simulink model "ASM_Traffic_V2X_Complete_Model_2"  (R2019a)
settings: Solver=ode1  StartTime=SIM.tstart.v  StopTime=Inf  FixedStep=SIM.StepSize.v  RelTol=1e-3
PostLoadFcn:
  | if any(exist('dsrtsu_mdlpostloadfcn', 'file') ~= 0), dsrtsu_mdlpostloadfcn('Execute', bdroot); end
  | try, asm_mdl_postloadfcn(bdroot, 'UpdateModel', 2200); catch, disp(lasterr); end,
undefined symbols (not defined in the file): _SensorPnts_1, _SensorPnts_13, _SensorPnts_17, _SensorPnts_21, _SensorPnts_25, _SensorPnts_29, _SensorPnts_33, _SensorPnts_37, _SensorPnts_41, _SensorPnts_45, _SensorPnts_49, _SensorPnts_5, _SensorPnts_53, _SensorPnts_57, _SensorPnts_9, _to_, CPT, G5A, ITS, MDL, rad, s_to_rpm, SIM
libraries: simulink x169, ASM_VehicleDynamics_lib x126, ASM_Traffic_lib x83, ASM_Utils_lib x49, mdbs x45, ASM_Environment_lib x17, dspindex x12, dsaV2xLibraryAux x10, dsmpblib x6, dsaV2xAsn1Library x4, dsaV2xLibrary x4, ASM_BrakeHydraulics_lib x4
(part 28 of 36)

== system ASM_Traffic_V2X_Complete_Model_2/MDLUserInterface/MotionDeskInterface/MOTION_DESK_INTERFACE/Traffic_Animation/Fellows_Animation/Fellow_11 ==
  Transform_In : Inport
  Pos_x_Fellows[m] : Inport  Port=2
  Pos_y_Fellows[m] : Inport  Port=3
  Pos_z_Fellows[m] : Inport  Port=4
  Angle_Roll_Fellows[deg] : Inport  Port=5
  Angle_Pitch_Fellows[deg] : Inport  Port=6
  Angle_Yaw_Fellows[deg] : Inport  Port=7
  Flag_FellowUsed : Inport  Port=8
  Constant : Constant  Value=11
  MD_Object : mdbs/MD_Object  strObjId=18  strObjName=Fellow_11  strBlockType=OBJ  bGUIEventOK=0
      settings: SourceProductName=dSPACE MotionDesk Blockset
  Mux : Mux  Inputs=3
  Mux1 : Mux  Inputs=3
  Mux3 : Mux  Inputs=3
  Selector{1..7} (7 alike) : Selector  InputPortWidth=MDL.Traffic.MaxNumFellows.v  IndexOptions=Index vector (port)  Indices=[1 3]  OutputSizes=1
  Terminator : Terminator
  wires:
  Pos_x_Fellows[m]/1 -> Selector1/1
  Pos_y_Fellows[m]/1 -> Selector2/1
  Pos_z_Fellows[m]/1 -> Selector3/1
  Angle_Roll_Fellows[deg]/1 -> Selector4/1
  Angle_Pitch_Fellows[deg]/1 -> Selector5/1
  Angle_Yaw_Fellows[deg]/1 -> Selector7/1
  Selector3/1 -> Mux/3
  Selector2/1 -> Mux/2
  Selector1/1 -> Mux/1
  Constant/1 -> Selector6/2, Selector7/2, Selector5/2, Selector4/2, Selector3/2, Selector2/2, Selector1/2
  Flag_FellowUsed/1 -> Selector6/1
  Mux1/1 -> MD_Object/3
  Mux3/1 -> MD_Object/4
  Transform_In/1 -> MD_Object/1
  Mux/1 -> MD_Object/2
  Selector6/1 -> Mux3/2, Mux3/3, Mux3/1
  MD_Object/1 -> Terminator/1
  Selector5/1 -> Mux1/2
  Selector7/1 -> Mux1/1
  Selector4/1 -> Mux1/3

== system ASM_Traffic_V2X_Complete_Model_2/MDLUserInterface/MotionDeskInterface/MOTION_DESK_INTERFACE/Traffic_Animation/Fellows_Animation/Fellow_12 ==
  Transform_In : Inport
  Pos_x_Fellows[m] : Inport  Port=2
  Pos_y_Fellows[m] : Inport  Port=3
  Pos_z_Fellows[m] : Inport  Port=4
  Angle_Roll_Fellows[deg] : Inport  Port=5
  Angle_Pitch_Fellows[deg] : Inport  Port=6
  Angle_Yaw_Fellows[deg] : Inport  Port=7
  Flag_FellowUsed : Inport  Port=8
  Constant : Constant  Value=12
  MD_Object : mdbs/MD_Object  strObjId=19  strObjName=Fellow_12  strBlockType=OBJ  bGUIEventOK=0
      settings: SourceProductName=dSPACE MotionDesk Blockset
  Mux : Mux  Inputs=3
  Mux1 : Mux  Inputs=3
  Mux3 : Mux  Inputs=3
  Selector{1..7} (7 alike) : Selector  InputPortWidth=MDL.Traffic.MaxNumFellows.v  IndexOptions=Index vector (port)  Indices=[1 3]  OutputSizes=1
  Terminator : Terminator
  wires:
  Pos_x_Fellows[m]/1 -> Selector1/1
  Pos_y_Fellows[m]/1 -> Selector2/1
  Pos_z_Fellows[m]/1 -> Selector3/1
  Angle_Roll_Fellows[deg]/1 -> Selector4/1
  Angle_Pitch_Fellows[deg]/1 -> Selector5/1
  Angle_Yaw_Fellows[deg]/1 -> Selector7/1
  Selector3/1 -> Mux/3
  Selector2/1 -> Mux/2
  Selector1/1 -> Mux/1
  Constant/1 -> Selector7/2, Selector6/2, Selector5/2, Selector4/2, Selector3/2, Selector2/2, Selector1/2
  Flag_FellowUsed/1 -> Selector6/1
  Mux1/1 -> MD_Object/3
  Mux3/1 -> MD_Object/4
  Transform_In/1 -> MD_Object/1
  Mux/1 -> MD_Object/2
  Selector6/1 -> Mux3/2, Mux3/3, Mux3/1
  MD_Object/1 -> Terminator/1
  Selector5/1 -> Mux1/2
  Selector7/1 -> Mux1/1
  Selector4/1 -> Mux1/3

== system ASM_Traffic_V2X_Complete_Model_2/MDLUserInterface/MotionDeskInterface/MOTION_DESK_INTERFACE/Traffic_Animation/Fellows_Animation/Fellow_13 ==
  Transform_In : Inport
  Pos_x_Fellows[m] : Inport  Port=2
  Pos_y_Fellows[m] : Inport  Port=3
  Pos_z_Fellows[m] : Inport  Port=4
  Angle_Roll_Fellows[deg] : Inport  Port=5
  Angle_Pitch_Fellows[deg] : Inport  Port=6
  Angle_Yaw_Fellows[deg] : Inport  Port=7
  Flag_FellowUsed : Inport  Port=8
  Constant : Constant  Value=13
  MD_Object : mdbs/MD_Object  strObjId=20  strObjName=Fellow_13  strBlockType=OBJ  bGUIEventOK=0
      settings: SourceProductName=dSPACE MotionDesk Blockset
  Mux : Mux  Inputs=3
  Mux1 : Mux  Inputs=3
  Mux3 : Mux  Inputs=3
  Selector{1..7} (7 alike) : Selector  InputPortWidth=MDL.Traffic.MaxNumFellows.v  IndexOptions=Index vector (port)  Indices=[1 3]  OutputSizes=1
  Terminator : Terminator
  wires:
  Pos_x_Fellows[m]/1 -> Selector1/1
  Pos_y_Fellows[m]/1 -> Selector2/1
  Pos_z_Fellows[m]/1 -> Selector3/1
  Angle_Roll_Fellows[deg]/1 -> Selector4/1
  Angle_Pitch_Fellows[deg]/1 -> Selector5/1
  Angle_Yaw_Fellows[deg]/1 -> Selector7/1
  Selector3/1 -> Mux/3
  Selector2/1 -> Mux/2
  Selector1/1 -> Mux/1
  Constant/1 -> Selector1/2, Selector6/2, Selector7/2, Selector5/2, Selector4/2, Selector3/2, Selector2/2
  Flag_FellowUsed/1 -> Selector6/1
  Mux1/1 -> MD_Object/3
  Mux3/1 -> MD_Object/4
  Transform_In/1 -> MD_Object/1
  Mux/1 -> MD_Object/2
  Selector6/1 -> Mux3/3, Mux3/2, Mux3/1
  MD_Object/1 -> Terminator/1
  Selector5/1 -> Mux1/2
  Selector7/1 -> Mux1/1
  Selector4/1 -> Mux1/3

== system ASM_Traffic_V2X_Complete_Model_2/MDLUserInterface/MotionDeskInterface/MOTION_DESK_INTERFACE/Traffic_Animation/Fellows_Animation/Fellow_14 ==
  Transform_In : Inport
  Pos_x_Fellows[m] : Inport  Port=2
  Pos_y_Fellows[m] : Inport  Port=3
  Pos_z_Fellows[m] : Inport  Port=4
  Angle_Roll_Fellows[deg] : Inport  Port=5
  Angle_Pitch_Fellows[deg] : Inport  Port=6
  Angle_Yaw_Fellows[deg] : Inport  Port=7
  Flag_FellowUsed : Inport  Port=8
  Constant : Constant  Value=14
  MD_Object : mdbs/MD_Object  strObjId=21  strObjName=Fellow_14  strBlockType=OBJ  bGUIEventOK=0
      settings: SourceProductName=dSPACE MotionDesk Blockset
  Mux : Mux  Inputs=3
  Mux1 : Mux  Inputs=3
  Mux3 : Mux  Inputs=3
  Selector{1..7} (7 alike) : Selector  InputPortWidth=MDL.Traffic.MaxNumFellows.v  IndexOptions=Index vector (port)  Indices=[1 3]  OutputSizes=1
  Terminator : Terminator
  wires:
  Pos_x_Fellows[m]/1 -> Selector1/1
  Pos_y_Fellows[m]/1 -> Selector2/1
  Pos_z_Fellows[m]/1 -> Selector3/1
  Angle_Roll_Fellows[deg]/1 -> Selector4/1
  Angle_Pitch_Fellows[deg]/1 -> Selector5/1
  Angle_Yaw_Fellows[deg]/1 -> Selector7/1
  Selector3/1 -> Mux/3
  Selector2/1 -> Mux/2
  Selector1/1 -> Mux/1
  Constant/1 -> Selector1/2, Selector6/2, Selector7/2, Selector5/2, Selector4/2, Selector3/2, Selector2/2
  Flag_FellowUsed/1 -> Selector6/1
  Mux1/1 -> MD_Object/3
  Mux3/1 -> MD_Object/4
  Transform_In/1 -> MD_Object/1
  Mux/1 -> MD_Object/2
  Selector6/1 -> Mux3/2, Mux3/3, Mux3/1
  MD_Object/1 -> Terminator/1
  Selector5/1 -> Mux1/2
  Selector7/1 -> Mux1/1
  Selector4/1 -> Mux1/3

== system ASM_Traffic_V2X_Complete_Model_2/MDLUserInterface/MotionDeskInterface/MOTION_DESK_INTERFACE/Traffic_Animation/Fellows_Animation/Fellow_15 ==
  Transform_In : Inport
  Pos_x_Fellows[m] : Inport  Port=2
  Pos_y_Fellows[m] : Inport  Port=3
  Pos_z_Fellows[m] : Inport  Port=4
  Angle_Roll_Fellows[deg] : Inport  Port=5
  Angle_Pitch_Fellows[deg] : Inport  Port=6
  Angle_Yaw_Fellows[deg] : Inport  Port=7
  Flag_FellowUsed : Inport  Port=8
  Constant : Constant  Value=15
  MD_Object : mdbs/MD_Object  strObjId=22  strObjName=Fellow_15  strBlockType=OBJ  bGUIEventOK=0
      settings: SourceProductName=dSPACE MotionDesk Blockset
  Mux : Mux  Inputs=3
  Mux1 : Mux  Inputs=3
  Mux3 : Mux  Inputs=3
  Selector{1..7} (7 alike) : Selector  InputPortWidth=MDL.Traffic.MaxNumFellows.v  IndexOptions=Index vector (port)  Indices=[1 3]  OutputSizes=1
  Terminator : Terminator
  wires:
  Pos_x_Fellows[m]/1 -> Selector1/1
  Pos_y_Fellows[m]/1 -> Selector2/1
  Pos_z_Fellows[m]/1 -> Selector3/1
  Angle_Roll_Fellows[deg]/1 -> Selector4/1
  Angle_Pitch_Fellows[deg]/1 -> Selector5/1
  Angle_Yaw_Fellows[deg]/1 -> Selector7/1
  Selector3/1 -> Mux/3
  Selector2/1 -> Mux/2
  Selector1/1 -> Mux/1
  Constant/1 -> Selector7/2, Selector6/2, Selector5/2, Selector4/2, Selector3/2, Selector2/2, Selector1/2
  Flag_FellowUsed/1 -> Selector6/1
  Mux1/1 -> MD_Object/3
  Mux3/1 -> MD_Object/4
  Transform_In/1 -> MD_Object/1
  Mux/1 -> MD_Object/2
  Selector6/1 -> Mux3/2, Mux3/3, Mux3/1
  MD_Object/1 -> Terminator/1
  Selector5/1 -> Mux1/2
  Selector7/1 -> Mux1/1
  Selector4/1 -> Mux1/3

== system ASM_Traffic_V2X_Complete_Model_2/MDLUserInterface/MotionDeskInterface/MOTION_DESK_INTERFACE/Traffic_Animation/Fellows_Animation/Fellow_2 ==
  Transform_In : Inport
  Pos_x_Fellows[m] : Inport  Port=2
  Pos_y_Fellows[m] : Inport  Port=3
  Pos_z_Fellows[m] : Inport  Port=4
  Angle_Roll_Fellows[deg] : Inport  Port=5
  Angle_Pitch_Fellows[deg] : Inport  Port=6
  Angle_Yaw_Fellows[deg] : Inport  Port=7
  Flag_FellowUsed : Inport  Port=8
  Constant : Constant  Value=2
  MD_Object : mdbs/MD_Object  strObjId=9  strObjName=Fellow_02  strBlockType=OBJ  bGUIEventOK=0
      settings: SourceProductName=dSPACE MotionDesk Blockset
  Mux : Mux  Inputs=3
  Mux1 : Mux  Inputs=3
  Mux3 : Mux  Inputs=3
  Selector{1..7} (7 alike) : Selector  InputPortWidth=MDL.Traffic.MaxNumFellows.v  IndexOptions=Index vector (port)  Indices=[1 3]  OutputSizes=1
  Terminator : Terminator
  wires:
  Pos_x_Fellows[m]/1 -> Selector1/1
  Pos_y_Fellows[m]/1 -> Selector2/1
  Pos_z_Fellows[m]/1 -> Selector3/1
  Angle_Roll_Fellows[deg]/1 -> Selector4/1
  Angle_Pitch_Fellows[deg]/1 -> Selector5/1
  Angle_Yaw_Fellows[deg]/1 -> Selector7/1
  Selector3/1 -> Mux/3
  Selector2/1 -> Mux/2
  Selector1/1 -> Mux/1
  Constant/1 -> Selector7/2, Selector6/2, Selector5/2, Selector4/2, Selector3/2, Selector2/2, Selector1/2
  Flag_FellowUsed/1 -> Selector6/1
  Mux3/1 -> MD_Object/4
  Transform_In/1 -> MD_Object/1
  Mux/1 -> MD_Object/2
  Mux1/1 -> MD_Object/3
  Selector6/1 -> Mux3/2, Mux3/3, Mux3/1
  MD_Object/1 -> Terminator/1
  Selector5/1 -> Mux1/2
  Selector7/1 -> Mux1/1
  Selector4/1 -> Mux1/3

== system ASM_Traffic_V2X_Complete_Model_2/MDLUserInterface/MotionDeskInterface/MOTION_DESK_INTERFACE/Traffic_Animation/Fellows_Animation/Fellow_3 ==
  Transform_In : Inport
  Pos_x_Fellows[m] : Inport  Port=2
  Pos_y_Fellows[m] : Inport  Port=3
  Pos_z_Fellows[m] : Inport  Port=4
  Angle_Roll_Fellows[deg] : Inport  Port=5
  Angle_Pitch_Fellows[deg] : Inport  Port=6
  Angle_Yaw_Fellows[deg] : Inport  Port=7
  Flag_FellowUsed : Inport  Port=8
  Constant : Constant  Value=3
  MD_Object : mdbs/MD_Object  strObjId=10  strObjName=Fellow_03  strBlockType=OBJ  bGUIEventOK=0
      settings: SourceProductName=dSPACE MotionDesk Blockset
  Mux : Mux  Inputs=3
  Mux1 : Mux  Inputs=3
  Mux3 : Mux  Inputs=3
  Selector{1..7} (7 alike) : Selector  InputPortWidth=MDL.Traffic.MaxNumFellows.v  IndexOptions=Index vector (port)  Indices=[1 3]  OutputSizes=1
  Terminator : Terminator
  wires:
  Selector4/1 -> Mux1/3
  Selector7/1 -> Mux1/1
  Selector5/1 -> Mux1/2
  MD_Object/1 -> Terminator/1
  Selector6/1 -> Mux3/1, Mux3/3, Mux3/2
  Mux1/1 -> MD_Object/3
  Mux/1 -> MD_Object/2
  Transform_In/1 -> MD_Object/1
  Mux3/1 -> MD_Object/4
  Flag_FellowUsed/1 -> Selector6/1
  Constant/1 -> Selector6/2, Selector7/2, Selector5/2, Selector4/2, Selector3/2, Selector2/2, Selector1/2
  Selector1/1 -> Mux/1
  Selector2/1 -> Mux/2
  Selector3/1 -> Mux/3
  Angle_Yaw_Fellows[deg]/1 -> Selector7/1
  Angle_Pitch_Fellows[deg]/1 -> Selector5/1
  Angle_Roll_Fellows[deg]/1 -> Selector4/1
  Pos_z_Fellows[m]/1 -> Selector3/1
  Pos_y_Fellows[m]/1 -> Selector2/1
  Pos_x_Fellows[m]/1 -> Selector1/1

== system ASM_Traffic_V2X_Complete_Model_2/MDLUserInterface/MotionDeskInterface/MOTION_DESK_INTERFACE/Traffic_Animation/Fellows_Animation/Fellow_4 ==
  Transform_In : Inport
  Pos_x_Fellows[m] : Inport  Port=2
  Pos_y_Fellows[m] : Inport  Port=3
  Pos_z_Fellows[m] : Inport  Port=4
  Angle_Roll_Fellows[deg] : Inport  Port=5
  Angle_Pitch_Fellows[deg] : Inport  Port=6
  Angle_Yaw_Fellows[deg] : Inport  Port=7
  Flag_FellowUsed : Inport  Port=8
  Constant : Constant  Value=4
  MD_Object : mdbs/MD_Object  strObjId=11  strObjName=Fellow_04  strBlockType=OBJ  bGUIEventOK=0
      settings: SourceProductName=dSPACE MotionDesk Blockset
  Mux : Mux  Inputs=3
  Mux1 : Mux  Inputs=3
  Mux3 : Mux  Inputs=3
  Selector{1..7} (7 alike) : Selector  InputPortWidth=MDL.Traffic.MaxNumFellows.v  IndexOptions=Index vector (port)  Indices=[1 3]  OutputSizes=1
  Terminator : Terminator
  wires:
  Pos_x_Fellows[m]/1 -> Selector1/1
  Pos_y_Fellows[m]/1 -> Selector2/1
  Pos_z_Fellows[m]/1 -> Selector3/1
  Angle_Roll_Fellows[deg]/1 -> Selector4/1
  Angle_Pitch_Fellows[deg]/1 -> Selector5/1
  Angle_Yaw_Fellows[deg]/1 -> Selector7/1
  Selector3/1 -> Mux/3
  Selector2/1 -> Mux/2
  Selector1/1 -> Mux/1
  Constant/1 -> Selector7/2, Selector6/2, Selector5/2, Selector4/2, Selector3/2, Selector2/2, Selector1/2
  Flag_FellowUsed/1 -> Selector6/1
  Mux3/1 -> MD_Object/4
  Transform_In/1 -> MD_Object/1
  Mux/1 -> MD_Object/2
  Mux1/1 -> MD_Object/3
  Selector6/1 -> Mux3/2, Mux3/3, Mux3/1
  MD_Object/1 -> Terminator/1
  Selector5/1 -> Mux1/2
  Selector7/1 -> Mux1/1
  Selector4/1 -> Mux1/3

== system ASM_Traffic_V2X_Complete_Model_2/MDLUserInterface/MotionDeskInterface/MOTION_DESK_INTERFACE/Traffic_Animation/Fellows_Animation/Fellow_5 ==
  Transform_In : Inport
  Pos_x_Fellows[m] : Inport  Port=2
  Pos_y_Fellows[m] : Inport  Port=3
  Pos_z_Fellows[m] : Inport  Port=4
  Angle_Roll_Fellows[deg] : Inport  Port=5
  Angle_Pitch_Fellows[deg] : Inport  Port=6
  Angle_Yaw_Fellows[deg] : Inport  Port=7
  Flag_FellowUsed : Inport  Port=8
  Constant : Constant  Value=5
  MD_Object : mdbs/MD_Object  strObjId=12  strObjName=Fellow_05  strBlockType=OBJ  bGUIEventOK=0
      settings: SourceProductName=dSPACE MotionDesk Blockset
  Mux : Mux  Inputs=3
  Mux1 : Mux  Inputs=3
  Mux3 : Mux  Inputs=3
  Selector{1..7} (7 alike) : Selector  InputPortWidth=MDL.Traffic.MaxNumFellows.v  IndexOptions=Index vector (port)  Indices=[1 3]  OutputSizes=1
  Terminator : Terminator
  wires:
  Pos_x_Fellows[m]/1 -> Selector1/1
  Pos_y_Fellows[m]/1 -> Selector2/1
  Pos_z_Fellows[m]/1 -> Selector3/1
  Angle_Roll_Fellows[deg]/1 -> Selector4/1
  Angle_Pitch_Fellows[deg]/1 -> Selector5/1
  Angle_Yaw_Fellows[deg]/1 -> Selector7/1
  Selector3/1 -> Mux/3
  Selector2/1 -> Mux/2
  Selector1/1 -> Mux/1
  Constant/1 -> Selector7/2, Selector6/2, Selector5/2, Selector4/2, Selector3/2, Selector2/2, Selector1/2
  Flag_FellowUsed/1 -> Selector6/1
  Mux1/1 -> MD_Object/3
  Mux3/1 -> MD_Object/4
  Transform_In/1 -> MD_Object/1
  Mux/1 -> MD_Object/2
  Selector6/1 -> Mux3/2, Mux3/3, Mux3/1
  MD_Object/1 -> Terminator/1
  Selector5/1 -> Mux1/2
  Selector7/1 -> Mux1/1
  Selector4/1 -> Mux1/3

== system ASM_Traffic_V2X_Complete_Model_2/MDLUserInterface/MotionDeskInterface/MOTION_DESK_INTERFACE/Traffic_Animation/Fellows_Animation/Fellow_6 ==
  Transform_In : Inport
  Pos_x_Fellows[m] : Inport  Port=2
  Pos_y_Fellows[m] : Inport  Port=3
  Pos_z_Fellows[m] : Inport  Port=4
  Angle_Roll_Fellows[deg] : Inport  Port=5
  Angle_Pitch_Fellows[deg] : Inport  Port=6
  Angle_Yaw_Fellows[deg] : Inport  Port=7
  Flag_FellowUsed : Inport  Port=8
  Constant : Constant  Value=6
  MD_Object : mdbs/MD_Object  strObjId=13  strObjName=Fellow_06  strBlockType=OBJ  bGUIEventOK=0
      settings: SourceProductName=dSPACE MotionDesk Blockset
  Mux : Mux  Inputs=3
  Mux1 : Mux  Inputs=3
  Mux3 : Mux  Inputs=3
  Selector{1..7} (7 alike) : Selector  InputPortWidth=MDL.Traffic.MaxNumFellows.v  IndexOptions=Index vector (port)  Indices=[1 3]  OutputSizes=1
  Terminator : Terminator
  wires:
  Pos_x_Fellows[m]/1 -> Selector1/1
  Pos_y_Fellows[m]/1 -> Selector2/1
  Pos_z_Fellows[m]/1 -> Selector3/1
  Angle_Roll_Fellows[deg]/1 -> Selector4/1
  Angle_Pitch_Fellows[deg]/1 -> Selector5/1
  Angle_Yaw_Fellows[deg]/1 -> Selector7/1
  Selector3/1 -> Mux/3
  Selector2/1 -> Mux/2
  Selector1/1 -> Mux/1
  Constant/1 -> Selector6/2, Selector7/2, Selector5/2, Selector4/2, Selector3/2, Selector2/2, Selector1/2
  Flag_FellowUsed/1 -> Selector6/1
  Mux1/1 -> MD_Object/3
  Mux3/1 -> MD_Object/4
  Transform_In/1 -> MD_Object/1
  Mux/1 -> MD_Object/2
  Selector6/1 -> Mux3/2, Mux3/3, Mux3/1
  MD_Object/1 -> Terminator/1
  Selector5/1 -> Mux1/2
  Selector7/1 -> Mux1/1
  Selector4/1 -> Mux1/3

== system ASM_Traffic_V2X_Complete_Model_2/MDLUserInterface/MotionDeskInterface/MOTION_DESK_INTERFACE/Traffic_Animation/Fellows_Animation/Fellow_7 ==
  Transform_In : Inport
  Pos_x_Fellows[m] : Inport  Port=2
  Pos_y_Fellows[m] : Inport  Port=3
  Pos_z_Fellows[m] : Inport  Port=4
  Angle_Roll_Fellows[deg] : Inport  Port=5
  Angle_Pitch_Fellows[deg] : Inport  Port=6
  Angle_Yaw_Fellows[deg] : Inport  Port=7
  Flag_FellowUsed : Inport  Port=8
  Constant : Constant  Value=7
  MD_Object : mdbs/MD_Object  strObjId=14  strObjName=Fellow_07  strBlockType=OBJ  bGUIEventOK=0
      settings: SourceProductName=dSPACE MotionDesk Blockset
  Mux : Mux  Inputs=3
  Mux1 : Mux  Inputs=3
  Mux3 : Mux  Inputs=3
  Selector{1..7} (7 alike) : Selector  InputPortWidth=MDL.Traffic.MaxNumFellows.v  IndexOptions=Index vector (port)  Indices=[1 3]  OutputSizes=1
  Terminator : Terminator
  wires:
  Pos_x_Fellows[m]/1 -> Selector1/1
  Pos_y_Fellows[m]/1 -> Selector2/1
  Pos_z_Fellows[m]/1 -> Selector3/1
  Angle_Roll_Fellows[deg]/1 -> Selector4/1
  Angle_Pitch_Fellows[deg]/1 -> Selector5/1
  Angle_Yaw_Fellows[deg]/1 -> Selector7/1
  Selector3/1 -> Mux/3
  Selector2/1 -> Mux/2
  Selector1/1 -> Mux/1
  Constant/1 -> Selector1/2, Selector7/2, Selector6/2, Selector5/2, Selector4/2, Selector3/2, Selector2/2
  Flag_FellowUsed/1 -> Selector6/1
  Mux1/1 -> MD_Object/3
  Mux3/1 -> MD_Object/4
  Transform_In/1 -> MD_Object/1
  Mux/1 -> MD_Object/2
  Selector6/1 -> Mux3/2, Mux3/3, Mux3/1
  MD_Object/1 -> Terminator/1
  Selector5/1 -> Mux1/2
  Selector7/1 -> Mux1/1
  Selector4/1 -> Mux1/3

== system ASM_Traffic_V2X_Complete_Model_2/MDLUserInterface/MotionDeskInterface/MOTION_DESK_INTERFACE/Traffic_Animation/Fellows_Animation/Fellow_8 ==
  Transform_In : Inport
  Pos_x_Fellows[m] : Inport  Port=2
  Pos_y_Fellows[m] : Inport  Port=3
  Pos_z_Fellows[m] : Inport  Port=4
  Angle_Roll_Fellows[deg] : Inport  Port=5
  Angle_Pitch_Fellows[deg] : Inport  Port=6
  Angle_Yaw_Fellows[deg] : Inport  Port=7
  Flag_FellowUsed : Inport  Port=8
  Constant : Constant  Value=8
  MD_Object : mdbs/MD_Object  strObjId=15  strObjName=Fellow_08  strBlockType=OBJ  bGUIEventOK=0
      settings: SourceProductName=dSPACE MotionDesk Blockset
  Mux : Mux  Inputs=3
  Mux1 : Mux  Inputs=3
  Mux3 : Mux  Inputs=3
  Selector{1..7} (7 alike) : Selector  InputPortWidth=MDL.Traffic.MaxNumFellows.v  IndexOptions=Index vector (port)  Indices=[1 3]  OutputSizes=1
  Terminator : Terminator
  wires:
  Pos_x_Fellows[m]/1 -> Selector1/1
  Pos_y_Fellows[m]/1 -> Selector2/1
  Pos_z_Fellows[m]/1 -> Selector3/1
  Angle_Roll_Fellows[deg]/1 -> Selector4/1
  Angle_Pitch_Fellows[deg]/1 -> Selector5/1
  Angle_Yaw_Fellows[deg]/1 -> Selector7/1
  Selector3/1 -> Mux/3
  Selector2/1 -> Mux/2
  Selector1/1 -> Mux/1
  Constant/1 -> Selector7/2, Selector6/2, Selector5/2, Selector4/2, Selector3/2, Selector2/2, Selector1/2
  Flag_FellowUsed/1 -> Selector6/1
  Mux1/1 -> MD_Object/3
  Mux3/1 -> MD_Object/4
  Transform_In/1 -> MD_Object/1
  Mux/1 -> MD_Object/2
  Selector6/1 -> Mux3/2, Mux3/3, Mux3/1
  MD_Object/1 -> Terminator/1
  Selector5/1 -> Mux1/2
  Selector7/1 -> Mux1/1
  Selector4/1 -> Mux1/3

== system ASM_Traffic_V2X_Complete_Model_2/MDLUserInterface/MotionDeskInterface/MOTION_DESK_INTERFACE/Traffic_Animation/Fellows_Animation/Fellow_9 ==
  Transform_In : Inport
  Pos_x_Fellows[m] : Inport  Port=2
  Pos_y_Fellows[m] : Inport  Port=3
  Pos_z_Fellows[m] : Inport  Port=4
  Angle_Roll_Fellows[deg] : Inport  Port=5
  Angle_Pitch_Fellows[deg] : Inport  Port=6
  Angle_Yaw_Fellows[deg] : Inport  Port=7
  Flag_FellowUsed : Inport  Port=8
  Constant : Constant  Value=9
  MD_Object : mdbs/MD_Object  strObjId=16  strObjName=Fellow_09  strBlockType=OBJ  bGUIEventOK=0
      settings: SourceProductName=dSPACE MotionDesk Blockset
  Mux : Mux  Inputs=3
  Mux1 : Mux  Inputs=3
  Mux3 : Mux  Inputs=3
  Selector{1..7} (7 alike) : Selector  InputPortWidth=MDL.Traffic.MaxNumFellows.v  IndexOptions=Index vector (port)  Indices=[1 3]  OutputSizes=1
  Terminator : Terminator
  wires:
  Pos_x_Fellows[m]/1 -> Selector1/1
  Pos_y_Fellows[m]/1 -> Selector2/1
  Pos_z_Fellows[m]/1 -> Selector3/1
  Angle_Roll_Fellows[deg]/1 -> Selector4/1
  Angle_Pitch_Fellows[deg]/1 -> Selector5/1
  Angle_Yaw_Fellows[deg]/1 -> Selector7/1
  Selector3/1 -> Mux/3
  Selector2/1 -> Mux/2
  Selector1/1 -> Mux/1
  Constant/1 -> Selector1/2, Selector6/2, Selector7/2, Selector5/2, Selector4/2, Selector3/2, Selector2/2
  Flag_FellowUsed/1 -> Selector6/1
  Mux1/1 -> MD_Object/3
  Mux3/1 -> MD_Object/4
  Transform_In/1 -> MD_Object/1
  Mux/1 -> MD_Object/2
  Selector6/1 -> Mux3/2, Mux3/3, Mux3/1
  MD_Object/1 -> Terminator/1
  Selector5/1 -> Mux1/2
  Selector7/1 -> Mux1/1
  Selector4/1 -> Mux1/3

== system ASM_Traffic_V2X_Complete_Model_2/MDLUserInterface/MotionDeskInterface/MOTION_DESK_INTERFACE/Traffic_Animation/Sensors_Animation/Sensor_Points ==
  Sw_Sensor_Animation[] : Inport
  Transform_In : Inport  Port=2
  Sensors_Signals : Inport  Port=3
  Bus Selector1 : BusSelector  OutputSignals=Object_Sensor_3D,Object_Sensor_2D,TrafficSign_Sensor_Dyn,Line_Sensor.Line_Sensor_1.Pos_Road_Lane_Animation_CoorSys_E,Line_Sensor.Line_Sensor_1.Pos_Road_Shape_Line_Animation_CoorSys_E,Line_Sensor.Line_Sensor_1.Pos_Road_Shape_ContObj_Animation_CoorSys_E,Line_Sensor.Line_Sensor_1.Pos_Junction_Border_Animation_CoorSys_E,Line_Sensor.Line_Sensor_1.Pos_Junction_Shape_Line_Animation_CoorSys_E,Line_Sensor.Line_Sensor_1.Pos_Junction_Shape_ContObj_Animation_CoorSys_E
  Line_Sensor_Junction_Border_Points : Subsystem
  Line_Sensor_Junction_Shape_ContObj_Points : Subsystem
  Line_Sensor_Junction_Shape_Line_Points : Subsystem
  Line_Sensor_Road_Lane_Points : Subsystem
  Line_Sensor_Road_Shape_ContObj_Points : Subsystem
  Line_Sensor_Road_Shape_Line_Points : Subsystem
  Multiport Switch : MultiPortSwitch  Inputs=11
  Object_Sensor_2D_Points : Subsystem
  Object_Sensor_3D_CustomPoints : Subsystem
  Object_Sensor_3D_Points : Subsystem
  Object_Sensor_3D_RadarEffect_Points : Subsystem
  Saturation : Saturate  UpperLimit=11  LowerLimit=1
  Sensor_Points : Subsystem
  Sensor_Selector : Constant
  Traffic_Sign_Sensor_Points : Subsystem
  wires:
  Sensor_Selector/1 -> Object_Sensor_3D_Points/2(Sensor_Selector), Object_Sensor_3D_CustomPoints/2(Sensor_Selector), Object_Sensor_3D_RadarEffect_Points/2(Sensor_Selector)
  Object_Sensor_3D_CustomPoints/1(AnimationSignals) -> Multiport Switch/12
  Object_Sensor_3D_RadarEffect_Points/1(AnimationSignals) -> Multiport Switch/11
  Bus Selector1/9 -> Line_Sensor_Junction_Shape_ContObj_Points/1(ModelSignals)  "<Pos_Junction_Shape_ContObj_Animation_CoorSys_E>"
  Line_Sensor_Junction_Shape_ContObj_Points/1(AnimationSignals) -> Multiport Switch/10
  Bus Selector1/8 -> Line_Sensor_Junction_Shape_Line_Points/1(ModelSignals)  "<Pos_Junction_Shape_Line_Animation_CoorSys_E>"
  Line_Sensor_Junction_Shape_Line_Points/1(AnimationSignals) -> Multiport Switch/9
  Sw_Sensor_Animation[]/1 -> Saturation/1
  Transform_In/1 -> Object_Sensor_2D_Points/1(Transform_In)
  Line_Sensor_Road_Lane_Points/1(AnimationSignals) -> Multiport Switch/5
  Traffic_Sign_Sensor_Points/1(AnimationSignals) -> Multiport Switch/4
  Object_Sensor_3D_Points/1(AnimationSignals) -> Multiport Switch/2
  Multiport Switch/1 -> Sensor_Points/1(AnimationSignals)
  Saturation/1 -> Multiport Switch/1
  Bus Selector1/3 -> Traffic_Sign_Sensor_Points/1(ModelSignals)  "<TrafficSign_Sensor_Dyn>"
  Bus Selector1/1 -> Object_Sensor_3D_Points/1(ModelSignals), Object_Sensor_3D_RadarEffect_Points/1(ModelSignals), Object_Sensor_3D_CustomPoints/1(ModelSignals)  "<Object_Sensor_3D>"
  Sensors_Signals/1 -> Bus Selector1/1
  Line_Sensor_Road_Shape_Line_Points/1(AnimationSignals) -> Multiport Switch/6
  Line_Sensor_Road_Shape_ContObj_Points/1(AnimationSignals) -> Multiport Switch/7
  Line_Sensor_Junction_Border_Points/1(AnimationSignals) -> Multiport Switch/8
  Bus Selector1/4 -> Line_Sensor_Road_Lane_Points/1(ModelSignals)  "<Pos_Road_Lane_Animation_CoorSys_E>"
  Bus Selector1/5 -> Line_Sensor_Road_Shape_Line_Points/1(ModelSignals)  "<Pos_Road_Shape_Line_Animation_CoorSys_E>"
  Bus Selector1/6 -> Line_Sensor_Road_Shape_ContObj_Points/1(ModelSignals)  "<Pos_Road_Shape_ContObj_Animation_CoorSys_E>"
  Bus Selector1/7 -> Line_Sensor_Junction_Border_Points/1(ModelSignals)  "<Pos_Junction_Border_Animation_CoorSys_E>"
  Bus Selector1/2 -> Object_Sensor_2D_Points/2(ModelSignals)  "<Object_Sensor_2D>"
  Object_Sensor_2D_Points/1(AnimationSignals) -> Multiport Switch/3

== system ASM_Traffic_V2X_Complete_Model_2/IO/I//O_Subsystem/Bus Configuration (1) - In/Simulated ECUs/DrivekitCAN/Drivekit/TX ==
  Input : Inport
  PDUs : Subsystem
  _TX_ : BusCreator  Inputs=1
  TX : Outport
  wires:
  _TX_/1 -> TX/1  "TX"
  PDUs/1(PDUs) -> _TX_/1  "PDUs"
  Input/1 -> PDUs/1(Input)

== system ASM_Traffic_V2X_Complete_Model_2/IO/I//O_Subsystem/Bus Configuration (1) - Out/Simulated ECUs/DrivekitCAN/Drivekit/RX ==
  RX : Inport
  PDUs : Subsystem
  _RX_ : BusSelector  OutputSignals=PDUs
  wires:
  RX/1 -> _RX_/1  "RX"
  _RX_/1 -> PDUs/1(PDUs)  "<PDUs>"

== system ASM_Traffic_V2X_Complete_Model_2/MDL/Drivetrain/Final_Drive_Assembly/ASMSignalCollector/FinalDrive_Ratio/FinalDriveRatio_FF_FF4WD/FinalDriveRatio[]_ ==
  In1 : Inport
  Out : Outport
  wires:
  In1/1 -> Out/1

== system ASM_Traffic_V2X_Complete_Model_2/MDL/Environment/Traffic/Sensors/Custom_Sensor/ASMSignalBus_Mapping/Combine1 ==
  Scopezone_In : Inport
  Values_In : Inport  Port=2
  Bus Creator1 : BusCreator  Inputs=13
  Bus Selector : BusSelector  OutputSignals=Object_ID[],Object_Type[],Pos_x_CoorSys_S[m],Pos_y_CoorSys_S[m],Pos_z_CoorSys_S[m],Angle_Hor_Rel[deg],Angle_Ver_Rel[deg],Distance[m],Network_Item_Type[0Junction|1Road],Network_Item_ID[],Parent_Object_ID[]
  Bus Selector1 : BusSelector  OutputSignals=Object_Valid[0|1],CustomValues[]
  Combined_Out : Outport
  wires:
  Bus Selector/11 -> Bus Creator1/12  "<Parent_Object_ID[]>"
  Bus Selector/10 -> Bus Creator1/11  "<Network_Item_ID[]>"
  Bus Selector/9 -> Bus Creator1/10  "<Network_Item_Type[0Junction|1Road]>"
  Bus Selector/8 -> Bus Creator1/9  "<Distance[m]>"
  Bus Selector/7 -> Bus Creator1/8  "<Angle_Ver_Rel[deg]>"
  Bus Selector/6 -> Bus Creator1/7  "<Angle_Hor_Rel[deg]>"
  Bus Selector/5 -> Bus Creator1/6  "<Pos_z_CoorSys_S[m]>"
  Bus Selector/4 -> Bus Creator1/5  "<Pos_y_CoorSys_S[m]>"
  Bus Selector/3 -> Bus Creator1/4  "<Pos_x_CoorSys_S[m]>"
  Bus Selector/2 -> Bus Creator1/3  "<Object_Type[]>"
  Bus Selector/1 -> Bus Creator1/2  "<Object_ID[]>"
  Bus Selector1/2 -> Bus Creator1/13  "<CustomValues[]>"
  Bus Selector1/1 -> Bus Creator1/1  "<Object_Valid[0|1]>"
  Values_In/1 -> Bus Selector1/1
  Scopezone_In/1 -> Bus Selector/1
  Bus Creator1/1 -> Combined_Out/1

== system ASM_Traffic_V2X_Complete_Model_2/MDL/Environment/Traffic/Sensors/Custom_Sensor/ASMSignalBus_Mapping/Combine2 ==
  Scopezone_In : Inport
  Values_In : Inport  Port=2
  Bus Creator1 : BusCreator  Inputs=13
  Bus Selector : BusSelector  OutputSignals=Object_ID[],Object_Type[],Pos_x_CoorSys_S[m],Pos_y_CoorSys_S[m],Pos_z_CoorSys_S[m],Angle_Hor_Rel[deg],Angle_Ver_Rel[deg],Distance[m],Network_Item_Type[0Junction|1Road],Network_Item_ID[],Parent_Object_ID[]
  Bus Selector1 : BusSelector  OutputSignals=Object_Valid[0|1],CustomValues[]
  Combined_Out : Outport
  wires:
  Bus Creator1/1 -> Combined_Out/1
  Scopezone_In/1 -> Bus Selector/1
  Values_In/1 -> Bus Selector1/1
  Bus Selector1/1 -> Bus Creator1/1  "<Object_Valid[0|1]>"
  Bus Selector1/2 -> Bus Creator1/13  "<CustomValues[]>"
  Bus Selector/1 -> Bus Creator1/2  "<Object_ID[]>"
  Bus Selector/2 -> Bus Creator1/3  "<Object_Type[]>"
  Bus Selector/3 -> Bus Creator1/4  "<Pos_x_CoorSys_S[m]>"
  Bus Selector/4 -> Bus Creator1/5  "<Pos_y_CoorSys_S[m]>"
  Bus Selector/5 -> Bus Creator1/6  "<Pos_z_CoorSys_S[m]>"
  Bus Selector/6 -> Bus Creator1/7  "<Angle_Hor_Rel[deg]>"
  Bus Selector/7 -> Bus Creator1/8  "<Angle_Ver_Rel[deg]>"
  Bus Selector/8 -> Bus Creator1/9  "<Distance[m]>"
  Bus Selector/9 -> Bus Creator1/10  "<Network_Item_Type[0Junction|1Road]>"
  Bus Selector/10 -> Bus Creator1/11  "<Network_Item_ID[]>"
  Bus Selector/11 -> Bus Creator1/12  "<Parent_Object_ID[]>"

== system ASM_Traffic_V2X_Complete_Model_2/MDL/Environment/Traffic/Sensors/Custom_Sensor/ASMSignalBus_Mapping/Combine3 ==
  Scopezone_In : Inport
  Values_In : Inport  Port=2
  Bus Creator1 : BusCreator  Inputs=13
  Bus Selector : BusSelector  OutputSignals=Object_ID[],Object_Type[],Pos_x_CoorSys_S[m],Pos_y_CoorSys_S[m],Pos_z_CoorSys_S[m],Angle_Hor_Rel[deg],Angle_Ver_Rel[deg],Distance[m],Network_Item_Type[0Junction|1Road],Network_Item_ID[],Parent_Object_ID[]
  Bus Selector1 : BusSelector  OutputSignals=Object_Valid[0|1],CustomValues[]
  Combined_Out : Outport
  wires:
  Bus Selector/11 -> Bus Creator1/12  "<Parent_Object_ID[]>"
  Bus Selector/10 -> Bus Creator1/11  "<Network_Item_ID[]>"
  Bus Selector/9 -> Bus Creator1/10  "<Network_Item_Type[0Junction|1Road]>"
  Bus Selector/8 -> Bus Creator1/9  "<Distance[m]>"
  Bus Selector/7 -> Bus Creator1/8  "<Angle_Ver_Rel[deg]>"
  Bus Selector/6 -> Bus Creator1/7  "<Angle_Hor_Rel[deg]>"
  Bus Selector/5 -> Bus Creator1/6  "<Pos_z_CoorSys_S[m]>"
  Bus Selector/4 -> Bus Creator1/5  "<Pos_y_CoorSys_S[m]>"
  Bus Selector/3 -> Bus Creator1/4  "<Pos_x_CoorSys_S[m]>"
  Bus Selector/2 -> Bus Creator1/3  "<Object_Type[]>"
  Bus Selector/1 -> Bus Creator1/2  "<Object_ID[]>"
  Bus Selector1/2 -> Bus Creator1/13  "<CustomValues[]>"
  Bus Selector1/1 -> Bus Creator1/1  "<Object_Valid[0|1]>"
  Values_In/1 -> Bus Selector1/1
  Scopezone_In/1 -> Bus Selector/1
  Bus Creator1/1 -> Combined_Out/1

== system ASM_Traffic_V2X_Complete_Model_2/MDL/Environment/Traffic/Sensors/Custom_Sensor/ASMSignalBus_Mapping/Combine4 ==
  Scopezone_In : Inport
  Values_In : Inport  Port=2
  Bus Creator1 : BusCreator  Inputs=13
  Bus Selector : BusSelector  OutputSignals=Object_ID[],Object_Type[],Pos_x_CoorSys_S[m],Pos_y_CoorSys_S[m],Pos_z_CoorSys_S[m],Angle_Hor_Rel[deg],Angle_Ver_Rel[deg],Distance[m],Network_Item_Type[0Junction|1Road],Network_Item_ID[],Parent_Object_ID[]
  Bus Selector1 : BusSelector  OutputSignals=Object_Valid[0|1],CustomValues[]
  Combined_Out : Outport
  wires:
  Bus Creator1/1 -> Combined_Out/1
  Scopezone_In/1 -> Bus Selector/1
  Values_In/1 -> Bus Selector1/1
  Bus Selector1/1 -> Bus Creator1/1  "<Object_Valid[0|1]>"
  Bus Selector1/2 -> Bus Creator1/13  "<CustomValues[]>"
  Bus Selector/1 -> Bus Creator1/2  "<Object_ID[]>"
  Bus Selector/2 -> Bus Creator1/3  "<Object_Type[]>"
  Bus Selector/3 -> Bus Creator1/4  "<Pos_x_CoorSys_S[m]>"
  Bus Selector/4 -> Bus Creator1/5  "<Pos_y_CoorSys_S[m]>"
  Bus Selector/5 -> Bus Creator1/6  "<Pos_z_CoorSys_S[m]>"
  Bus Selector/6 -> Bus Creator1/7  "<Angle_Hor_Rel[deg]>"
  Bus Selector/7 -> Bus Creator1/8  "<Angle_Ver_Rel[deg]>"
  Bus Selector/8 -> Bus Creator1/9  "<Distance[m]>"
  Bus Selector/9 -> Bus Creator1/10  "<Network_Item_Type[0Junction|1Road]>"
  Bus Selector/10 -> Bus Creator1/11  "<Network_Item_ID[]>"
  Bus Selector/11 -> Bus Creator1/12  "<Parent_Object_ID[]>"

== system ASM_Traffic_V2X_Complete_Model_2/MDL/Environment/Traffic/Sensors/Custom_Sensor/ASMSignalBus_Mapping/Combine5 ==
  Scopezone_In : Inport
  Values_In : Inport  Port=2
  Bus Creator1 : BusCreator  Inputs=13
  Bus Selector : BusSelector  OutputSignals=Object_ID[],Object_Type[],Pos_x_CoorSys_S[m],Pos_y_CoorSys_S[m],Pos_z_CoorSys_S[m],Angle_Hor_Rel[deg],Angle_Ver_Rel[deg],Distance[m],Network_Item_Type[0Junction|1Road],Network_Item_ID[],Parent_Object_ID[]
  Bus Selector1 : BusSelector  OutputSignals=Object_Valid[0|1],CustomValues[]
  Combined_Out : Outport
  wires:
  Bus Selector/11 -> Bus Creator1/12  "<Parent_Object_ID[]>"
  Bus Selector/10 -> Bus Creator1/11  "<Network_Item_ID[]>"
  Bus Selector/9 -> Bus Creator1/10  "<Network_Item_Type[0Junction|1Road]>"
  Bus Selector/8 -> Bus Creator1/9  "<Distance[m]>"
  Bus Selector/7 -> Bus Creator1/8  "<Angle_Ver_Rel[deg]>"
  Bus Selector/6 -> Bus Creator1/7  "<Angle_Hor_Rel[deg]>"
  Bus Selector/5 -> Bus Creator1/6  "<Pos_z_CoorSys_S[m]>"
  Bus Selector/4 -> Bus Creator1/5  "<Pos_y_CoorSys_S[m]>"
  Bus Selector/3 -> Bus Creator1/4  "<Pos_x_CoorSys_S[m]>"
  Bus Selector/2 -> Bus Creator1/3  "<Object_Type[]>"
  Bus Selector/1 -> Bus Creator1/2  "<Object_ID[]>"
  Bus Selector1/2 -> Bus Creator1/13  "<CustomValues[]>"
  Bus Selector1/1 -> Bus Creator1/1  "<Object_Valid[0|1]>"
  Values_In/1 -> Bus Selector1/1
  Scopezone_In/1 -> Bus Selector/1
  Bus Creator1/1 -> Combined_Out/1

== system ASM_Traffic_V2X_Complete_Model_2/MDL/Environment/Traffic/Sensors/Custom_Sensor/ASMSignalBus_Mapping/CombineInfo ==
  Scopezone_In : Inport
  Values_In : Inport  Port=2
  Bus Creator1 : BusCreator  Inputs=3
  Bus Selector : BusSelector  OutputSignals=CustomSensor_ScopezoneSfcn_State[],CustomSensor_ScopezoneSfcn_Data_Valid[0|1]
  Bus Selector1 : BusSelector  OutputSignals=CustomSensor_OutputSfcn_State[],CustomSensor_OutputSfcn_Data_Valid[0|1]
  Product : Product  RndMeth=Zero
  Combined_Out : Outport
  wires:
  Product/1 -> Bus Creator1/3  "CustomSensor_Data_Valid[0|1]"
  Bus Selector1/2 -> Product/2  "<CustomSensor_OutputSfcn_Data_Valid[0|1]>"
  Bus Selector1/1 -> Bus Creator1/2  "<CustomSensor_OutputSfcn_State[]>"
  Bus Selector/2 -> Product/1  "<CustomSensor_ScopezoneSfcn_Data_Valid[0|1]>"
  Bus Selector/1 -> Bus Creator1/1  "<CustomSensor_ScopezoneSfcn_State[]>"
  Bus Creator1/1 -> Combined_Out/1
  Scopezone_In/1 -> Bus Selector/1
  Values_In/1 -> Bus Selector1/1

== system ASM_Traffic_V2X_Complete_Model_2/MDL/Environment/Traffic/Sensors/Custom_Sensor/SensorOutput_Mapping/Combine1 ==
  Scopezone_In : Inport
  Values_In : Inport  Port=2
  Bus Creator1 : BusCreator  Inputs=13
  Bus Selector : BusSelector  OutputSignals=Object_ID[],Object_Type[],Pos_x_CoorSys_S[m],Pos_y_CoorSys_S[m],Pos_z_CoorSys_S[m],Angle_Hor_Rel[deg],Angle_Ver_Rel[deg],Distance[m],Network_Item_Type[0Junction|1Road],Network_Item_ID[],Parent_Object_ID[]
  Bus Selector1 : BusSelector  OutputSignals=Object_Valid[0|1],CustomValues[]
  Combined_Out : Outport
  wires:
  Bus Selector/11 -> Bus Creator1/12  "<Parent_Object_ID[]>"
  Bus Selector/10 -> Bus Creator1/11  "<Network_Item_ID[]>"
  Bus Selector/9 -> Bus Creator1/10  "<Network_Item_Type[0Junction|1Road]>"
  Bus Selector/8 -> Bus Creator1/9  "<Distance[m]>"
  Bus Selector/7 -> Bus Creator1/8  "<Angle_Ver_Rel[deg]>"
  Bus Selector/6 -> Bus Creator1/7  "<Angle_Hor_Rel[deg]>"
  Bus Selector/5 -> Bus Creator1/6  "<Pos_z_CoorSys_S[m]>"
  Bus Selector/4 -> Bus Creator1/5  "<Pos_y_CoorSys_S[m]>"
  Bus Selector/3 -> Bus Creator1/4  "<Pos_x_CoorSys_S[m]>"
  Bus Selector/2 -> Bus Creator1/3  "<Object_Type[]>"
  Bus Selector/1 -> Bus Creator1/2  "<Object_ID[]>"
  Bus Selector1/2 -> Bus Creator1/13  "<CustomValues[]>"
  Bus Selector1/1 -> Bus Creator1/1  "<Object_Valid[0|1]>"
  Values_In/1 -> Bus Selector1/1
  Scopezone_In/1 -> Bus Selector/1
  Bus Creator1/1 -> Combined_Out/1

== system ASM_Traffic_V2X_Complete_Model_2/MDL/Environment/Traffic/Sensors/Custom_Sensor/SensorOutput_Mapping/Combine2 ==
  Scopezone_In : Inport
  Values_In : Inport  Port=2
  Bus Creator1 : BusCreator  Inputs=13
  Bus Selector : BusSelector  OutputSignals=Object_ID[],Object_Type[],Pos_x_CoorSys_S[m],Pos_y_CoorSys_S[m],Pos_z_CoorSys_S[m],Angle_Hor_Rel[deg],Angle_Ver_Rel[deg],Distance[m],Network_Item_Type[0Junction|1Road],Network_Item_ID[],Parent_Object_ID[]
  Bus Selector1 : BusSelector  OutputSignals=Object_Valid[0|1],CustomValues[]
  Combined_Out : Outport
  wires:
  Bus Creator1/1 -> Combined_Out/1
  Scopezone_In/1 -> Bus Selector/1
  Values_In/1 -> Bus Selector1/1
  Bus Selector1/1 -> Bus Creator1/1  "<Object_Valid[0|1]>"
  Bus Selector1/2 -> Bus Creator1/13  "<CustomValues[]>"
  Bus Selector/1 -> Bus Creator1/2  "<Object_ID[]>"
  Bus Selector/2 -> Bus Creator1/3  "<Object_Type[]>"
  Bus Selector/3 -> Bus Creator1/4  "<Pos_x_CoorSys_S[m]>"
  Bus Selector/4 -> Bus Creator1/5  "<Pos_y_CoorSys_S[m]>"
  Bus Selector/5 -> Bus Creator1/6  "<Pos_z_CoorSys_S[m]>"
  Bus Selector/6 -> Bus Creator1/7  "<Angle_Hor_Rel[deg]>"
  Bus Selector/7 -> Bus Creator1/8  "<Angle_Ver_Rel[deg]>"
  Bus Selector/8 -> Bus Creator1/9  "<Distance[m]>"
  Bus Selector/9 -> Bus Creator1/10  "<Network_Item_Type[0Junction|1Road]>"
  Bus Selector/10 -> Bus Creator1/11  "<Network_Item_ID[]>"
  Bus Selector/11 -> Bus Creator1/12  "<Parent_Object_ID[]>"

== system ASM_Traffic_V2X_Complete_Model_2/MDL/Environment/Traffic/Sensors/Custom_Sensor/SensorOutput_Mapping/Combine3 ==
  Scopezone_In : Inport
  Values_In : Inport  Port=2
  Bus Creator1 : BusCreator  Inputs=13
  Bus Selector : BusSelector  OutputSignals=Object_ID[],Object_Type[],Pos_x_CoorSys_S[m],Pos_y_CoorSys_S[m],Pos_z_CoorSys_S[m],Angle_Hor_Rel[deg],Angle_Ver_Rel[deg],Distance[m],Network_Item_Type[0Junction|1Road],Network_Item_ID[],Parent_Object_ID[]
  Bus Selector1 : BusSelector  OutputSignals=Object_Valid[0|1],CustomValues[]
  Combined_Out : Outport
  wires:
  Bus Selector/11 -> Bus Creator1/12  "<Parent_Object_ID[]>"
  Bus Selector/10 -> Bus Creator1/11  "<Network_Item_ID[]>"
  Bus Selector/9 -> Bus Creator1/10  "<Network_Item_Type[0Junction|1Road]>"
  Bus Selector/8 -> Bus Creator1/9  "<Distance[m]>"
  Bus Selector/7 -> Bus Creator1/8  "<Angle_Ver_Rel[deg]>"
  Bus Selector/6 -> Bus Creator1/7  "<Angle_Hor_Rel[deg]>"
  Bus Selector/5 -> Bus Creator1/6  "<Pos_z_CoorSys_S[m]>"
  Bus Selector/4 -> Bus Creator1/5  "<Pos_y_CoorSys_S[m]>"
  Bus Selector/3 -> Bus Creator1/4  "<Pos_x_CoorSys_S[m]>"
  Bus Selector/2 -> Bus Creator1/3  "<Object_Type[]>"
  Bus Selector/1 -> Bus Creator1/2  "<Object_ID[]>"
  Bus Selector1/2 -> Bus Creator1/13  "<CustomValues[]>"
  Bus Selector1/1 -> Bus Creator1/1  "<Object_Valid[0|1]>"
  Values_In/1 -> Bus Selector1/1
  Scopezone_In/1 -> Bus Selector/1
  Bus Creator1/1 -> Combined_Out/1

== system ASM_Traffic_V2X_Complete_Model_2/MDL/Environment/Traffic/Sensors/Custom_Sensor/SensorOutput_Mapping/Combine4 ==
  Scopezone_In : Inport
  Values_In : Inport  Port=2
  Bus Creator1 : BusCreator  Inputs=13
  Bus Selector : BusSelector  OutputSignals=Object_ID[],Object_Type[],Pos_x_CoorSys_S[m],Pos_y_CoorSys_S[m],Pos_z_CoorSys_S[m],Angle_Hor_Rel[deg],Angle_Ver_Rel[deg],Distance[m],Network_Item_Type[0Junction|1Road],Network_Item_ID[],Parent_Object_ID[]
  Bus Selector1 : BusSelector  OutputSignals=Object_Valid[0|1],CustomValues[]
  Combined_Out : Outport
  wires:
  Bus Creator1/1 -> Combined_Out/1
  Scopezone_In/1 -> Bus Selector/1
  Values_In/1 -> Bus Selector1/1
  Bus Selector1/1 -> Bus Creator1/1  "<Object_Valid[0|1]>"
  Bus Selector1/2 -> Bus Creator1/13  "<CustomValues[]>"
  Bus Selector/1 -> Bus Creator1/2  "<Object_ID[]>"
  Bus Selector/2 -> Bus Creator1/3  "<Object_Type[]>"
  Bus Selector/3 -> Bus Creator1/4  "<Pos_x_CoorSys_S[m]>"
  Bus Selector/4 -> Bus Creator1/5  "<Pos_y_CoorSys_S[m]>"
  Bus Selector/5 -> Bus Creator1/6  "<Pos_z_CoorSys_S[m]>"
  Bus Selector/6 -> Bus Creator1/7  "<Angle_Hor_Rel[deg]>"
  Bus Selector/7 -> Bus Creator1/8  "<Angle_Ver_Rel[deg]>"
  Bus Selector/8 -> Bus Creator1/9  "<Distance[m]>"
  Bus Selector/9 -> Bus Creator1/10  "<Network_Item_Type[0Junction|1Road]>"
  Bus Selector/10 -> Bus Creator1/11  "<Network_Item_ID[]>"
  Bus Selector/11 -> Bus Creator1/12  "<Parent_Object_ID[]>"

== system ASM_Traffic_V2X_Complete_Model_2/MDL/Environment/Traffic/Sensors/Custom_Sensor/SensorOutput_Mapping/Combine5 ==
  Scopezone_In : Inport
  Values_In : Inport  Port=2
  Bus Creator1 : BusCreator  Inputs=13
  Bus Selector : BusSelector  OutputSignals=Object_ID[],Object_Type[],Pos_x_CoorSys_S[m],Pos_y_CoorSys_S[m],Pos_z_CoorSys_S[m],Angle_Hor_Rel[deg],Angle_Ver_Rel[deg],Distance[m],Network_Item_Type[0Junction|1Road],Network_Item_ID[],Parent_Object_ID[]
  Bus Selector1 : BusSelector  OutputSignals=Object_Valid[0|1],CustomValues[]
  Combined_Out : Outport
  wires:
  Bus Selector/11 -> Bus Creator1/12  "<Parent_Object_ID[]>"
  Bus Selector/10 -> Bus Creator1/11  "<Network_Item_ID[]>"
  Bus Selector/9 -> Bus Creator1/10  "<Network_Item_Type[0Junction|1Road]>"
  Bus Selector/8 -> Bus Creator1/9  "<Distance[m]>"
  Bus Selector/7 -> Bus Creator1/8  "<Angle_Ver_Rel[deg]>"
  Bus Selector/6 -> Bus Creator1/7  "<Angle_Hor_Rel[deg]>"
  Bus Selector/5 -> Bus Creator1/6  "<Pos_z_CoorSys_S[m]>"
  Bus Selector/4 -> Bus Creator1/5  "<Pos_y_CoorSys_S[m]>"
  Bus Selector/3 -> Bus Creator1/4  "<Pos_x_CoorSys_S[m]>"
  Bus Selector/2 -> Bus Creator1/3  "<Object_Type[]>"
  Bus Selector/1 -> Bus Creator1/2  "<Object_ID[]>"
  Bus Selector1/2 -> Bus Creator1/13  "<CustomValues[]>"
  Bus Selector1/1 -> Bus Creator1/1  "<Object_Valid[0|1]>"
  Values_In/1 -> Bus Selector1/1
  Scopezone_In/1 -> Bus Selector/1
  Bus Creator1/1 -> Combined_Out/1

== system ASM_Traffic_V2X_Complete_Model_2/MDL/Environment/Traffic/Sensors/Object_Sensor_2D/ScheduleAndCalculateSensor/SampleAndHold ==
  In1 : Inport
  In2 : Inport  Port=2
  In3 : Inport  Port=3
  In4 : Inport  Port=4
  In5 : Inport  Port=5
  Enable : EnablePort
  Out1 : Outport
  Out2 : Outport  Port=2
  Out3 : Outport  Port=3
  Out4 : Outport  Port=4
  Out5 : Outport  Port=5
  wires:
  In5/1 -> Out5/1
  In4/1 -> Out4/1
  In3/1 -> Out3/1
  In1/1 -> Out1/1
  In2/1 -> Out2/1

== system ASM_Traffic_V2X_Complete_Model_2/MDL/Environment/Traffic/Sensors/Object_Sensor_3D/CustomPoints/Sensor1 ==
  Enable[0|1] : Inport
  SensorMapping_Data[] : Inport  Port=2
  SensorData[] : Inport  Port=3
  CustomPoints : Subsystem
  CustomPointsOutput : Subsystem
  Demux : Demux
  CustomPoints_Signals[] : Outport
  wires:
  CustomPointsOutput/1(CustomPoints_Signals_Out[]) -> CustomPoints_Signals[]/1
  CustomPoints/1(CustomPoint_Signals[]) -> CustomPointsOutput/5(CustomPoints_Signals_In[])
  Enable[0|1]/1 -> CustomPointsOutput/1(SensorSchedulingEnable[0|1])
  Demux/3 -> CustomPointsOutput/4(DelayPulse[0|1])
  Demux/2 -> CustomPointsOutput/3(SensorEnable[0|1]), CustomPoints/Enable
  Demux/1 -> CustomPointsOutput/2(SensorActive[0|1])
  Demux/4 -> CustomPoints/1(Sensor_Idx[])
  SensorData[]/1 -> CustomPoints/2(Sensor_Data[])
  SensorMapping_Data[]/1 -> Demux/1

== system ASM_Traffic_V2X_Complete_Model_2/MDL/Environment/Traffic/Sensors/Object_Sensor_3D/CustomPoints/Sensor2 ==
  Enable[0|1] : Inport
  SensorMapping_Data[] : Inport  Port=2
  SensorData[] : Inport  Port=3
  CustomPoints : Subsystem
  CustomPointsOutput : Subsystem
  Demux : Demux
  CustomPoints_Signals[] : Outport
  wires:
  Demux/3 -> CustomPointsOutput/4(DelayPulse[0|1])
  Demux/2 -> CustomPoints/Enable, CustomPointsOutput/3(SensorEnable[0|1])
  CustomPointsOutput/1(CustomPoints_Signals_Out[]) -> CustomPoints_Signals[]/1
  CustomPoints/1(CustomPoint_Signals[]) -> CustomPointsOutput/5(CustomPoint_Signals_In[])
  Demux/1 -> CustomPointsOutput/2(SensorActive[0|1])
  Demux/4 -> CustomPoints/1(Sensor_Idx[])
  SensorData[]/1 -> CustomPoints/2(Sensor_Data[])
  Enable[0|1]/1 -> CustomPointsOutput/1(SensorSchedulingEnable[0|1])
  SensorMapping_Data[]/1 -> Demux/1

== system ASM_Traffic_V2X_Complete_Model_2/MDL/Environment/Traffic/Sensors/Object_Sensor_3D/CustomPoints/Sensor3 ==
  Enable[0|1] : Inport
  SensorMapping_Data[] : Inport  Port=2
  SensorData[] : Inport  Port=3
  CustomPoints : Subsystem
  CustomPointsOutput : Subsystem
  Demux : Demux
  CustomPoints_Signals[] : Outport
  wires:
  Demux/3 -> CustomPointsOutput/4(DelayPulse[0|1])
  Demux/2 -> CustomPoints/Enable, CustomPointsOutput/3(SensorEnable[0|1])
  Demux/1 -> CustomPointsOutput/2(SensorActive[0|1])
  CustomPoints/1(CustomPoint_Signals[]) -> CustomPointsOutput/5(CustomPoints_Signals_In[])
  CustomPointsOutput/1(CustomPoints_Signals_Out[]) -> CustomPoints_Signals[]/1
  Enable[0|1]/1 -> CustomPointsOutput/1(SensorSchedulingEnable[0|1])
  Demux/4 -> CustomPoints/1(Sensor_Idx[])
  SensorData[]/1 -> CustomPoints/2(Sensor_Data[])
  SensorMapping_Data[]/1 -> Demux/1

== system ASM_Traffic_V2X_Complete_Model_2/MDL/Environment/Traffic/Sensors/Object_Sensor_3D/RadarEffects/Sensor1 ==
  Enable[0|1] : Inport
  SensorMapping_Data[] : Inport  Port=2
  Sensor_Data[] : Inport  Port=3
  Angle_Vehicle_CoorSys_E[x;y;z][deg] : Inport  Port=4
  Pos_Vehicle_CoorSys_E[x;y;z][m] : Inport  Port=5
  Bus Selector : BusSelector  OutputSignals=Angle_Orientation_Sensor_CoorSys_V[x;y;z][deg],Pos_Sensor_Apex_CoorSys_V[x;y;z][m]
  Demux : Demux
  RadarEffects : Subsystem
  RadarEffectsOutput : Subsystem
  RadarEffect_Signals[] : Outport
  wires:
  RadarEffectsOutput/1(RadarEffect_Signals_Out[]) -> RadarEffect_Signals[]/1
  RadarEffects/1(RadarEffect_Signals[]) -> RadarEffectsOutput/5(RadarEffect_Signals_In[])
  Demux/3 -> RadarEffectsOutput/4(DelayPulse[0|1])
  Enable[0|1]/1 -> RadarEffectsOutput/1(SensorSchedulingEnable[0|1])
  Demux/2 -> RadarEffectsOutput/3(SensorEnable[0|1]), RadarEffects/Enable
  Demux/1 -> RadarEffectsOutput/2(SensorActive[0|1])
  SensorMapping_Data[]/1 -> Demux/1
  [ASMBUS_Environment_Traffic_3DObjSensor1_Parameters] -> Bus Selector/1
  Bus Selector/1 -> RadarEffects/5(Angle_Sensor_CoorSys_V[x;y;z][deg])  "<Angle_Orientation_Sensor_CoorSys_V[x;y;z][deg]>"
  Bus Selector/2 -> RadarEffects/6(Pos_Sensor_CoorSys_V[x;y;z][m])  "<Pos_Sensor_Apex_CoorSys_V[x;y;z][m]>"
  Pos_Vehicle_CoorSys_E[x;y;z][m]/1 -> RadarEffects/4(Pos_Vehicle_CoorSys_E[x;y;z][m])
  Sensor_Data[]/1 -> RadarEffects/2(Sensor_Data[])
  Angle_Vehicle_CoorSys_E[x;y;z][deg]/1 -> RadarEffects/3(Angle_Vehicle_CoorSys_E[x;y;z][deg])
  Demux/4 -> RadarEffects/1(Sensor_Idx[])

== system ASM_Traffic_V2X_Complete_Model_2/MDL/Environment/Traffic/Sensors/Object_Sensor_3D/RadarEffects/Sensor2 ==
  Enable[0|1] : Inport
  SensorMapping_Data[] : Inport  Port=2
  Sensor_Data[] : Inport  Port=3
  Angle_Vehicle_CoorSys_E[x;y;z][deg] : Inport  Port=4
  Pos_Vehicle_CoorSys_E[x;y;z][m] : Inport  Port=5
  Bus Selector : BusSelector  OutputSignals=Angle_Orientation_Sensor_CoorSys_V[x;y;z][deg],Pos_Sensor_Apex_CoorSys_V[x;y;z][m]
  Demux : Demux
  RadarEffects : Subsystem
  RadarEffectsOutput : Subsystem
  RadarEffect_Signals[] : Outport
  wires:
  Demux/2 -> RadarEffectsOutput/3(SensorEnable[0|1]), RadarEffects/Enable
  RadarEffectsOutput/1(RadarEffect_Signals_Out[]) -> RadarEffect_Signals[]/1
  RadarEffects/1(RadarEffect_Signals[]) -> RadarEffectsOutput/5(RadarEffect_Signals_In[])
  Enable[0|1]/1 -> RadarEffectsOutput/1(SensorScheudlingEnable[0|1])
  Demux/3 -> RadarEffectsOutput/4(DelayPulse[0|1])
  Demux/1 -> RadarEffectsOutput/2(SensorActive)
  SensorMapping_Data[]/1 -> Demux/1
  [ASMBUS_Environment_Traffic_3DObjSensor2_Parameters] -> Bus Selector/1
  Bus Selector/1 -> RadarEffects/5(Angle_Sensor_CoorSys_V[x;y;z][deg])  "<Angle_Orientation_Sensor_CoorSys_V[x;y;z][deg]>"
  Bus Selector/2 -> RadarEffects/6(Pos_Sensor_CoorSys_V[x;y;z][m])  "<Pos_Sensor_Apex_CoorSys_V[x;y;z][m]>"
  Pos_Vehicle_CoorSys_E[x;y;z][m]/1 -> RadarEffects/4(Pos_Vehicle_CoorSys_E[x;y;z][m])
  Sensor_Data[]/1 -> RadarEffects/2(Sensor_Data[])
  Angle_Vehicle_CoorSys_E[x;y;z][deg]/1 -> RadarEffects/3(Angle_Vehicle_CoorSys_E[x;y;z][deg])
  Demux/4 -> RadarEffects/1(Sensor_Idx[])

== system ASM_Traffic_V2X_Complete_Model_2/MDL/Environment/Traffic/Sensors/Object_Sensor_3D/RadarEffects/Sensor3 ==
  Enable[0|1] : Inport
  SensorMapping_Data[] : Inport  Port=2
  Sensor_Data[] : Inport  Port=3
  Angle_Vehicle_CoorSys_E[x;y;z][deg] : Inport  Port=4
  Pos_Vehicle_CoorSys_E[x;y;z][m] : Inport  Port=5
  Bus Selector : BusSelector  OutputSignals=Angle_Orientation_Sensor_CoorSys_V[x;y;z][deg],Pos_Sensor_Apex_CoorSys_V[x;y;z][m]
  Demux : Demux
  RadarEffects : Subsystem
  RadarEffectsOutput : Subsystem
  RadarEffect_Signals[] : Outport
  wires:
  Demux/2 -> RadarEffects/Enable, RadarEffectsOutput/3(SensorEnable[0|1])
  RadarEffectsOutput/1(RadarEffect_Signals_Out[]) -> RadarEffect_Signals[]/1
  RadarEffects/1(RadarEffect_Signals[]) -> RadarEffectsOutput/5(RadarEffect_Signals_In[])
  Enable[0|1]/1 -> RadarEffectsOutput/1(SensorSchedulingEnable[0|1])
  Demux/3 -> RadarEffectsOutput/4(DelayPulse[0|1])
  Demux/4 -> RadarEffects/1(Sensor_Idx[])
  Angle_Vehicle_CoorSys_E[x;y;z][deg]/1 -> RadarEffects/3(Angle_Vehicle_CoorSys_E[x;y;z][deg])
  Sensor_Data[]/1 -> RadarEffects/2(Sensor_Data[])
  Pos_Vehicle_CoorSys_E[x;y;z][m]/1 -> RadarEffects/4(Pos_Vehicle_CoorSys_E[x;y;z][m])
  Bus Selector/2 -> RadarEffects/6(Pos_Sensor_CoorSys_V[x;y;z][m])  "<Pos_Sensor_Apex_CoorSys_V[x;y;z][m]>"
  Bus Selector/1 -> RadarEffects/5(Angle_Sensor_CoorSys_V[x;y;z][deg])  "<Angle_Orientation_Sensor_CoorSys_V[x;y;z][deg]>"
  [ASMBUS_Environment_Traffic_3DObjSensor3_Parameters] -> Bus Selector/1
  SensorMapping_Data[]/1 -> Demux/1
  Demux/1 -> RadarEffectsOutput/2(SensorActive[0|1])

== system ASM_Traffic_V2X_Complete_Model_2/MDL/Environment/Traffic/Sensors/Object_Sensor_3D/ScheduleAndCalculateSensor/SampleAndHold ==
  In1 : Inport
  In2 : Inport  Port=2
  In3 : Inport  Port=3
  In4 : Inport  Port=4
  In5 : Inport  Port=5
  Enable : EnablePort
  Out1 : Outport
  Out2 : Outport  Port=2
  Out3 : Outport  Port=3
  Out4 : Outport  Port=4
  Out5 : Outport  Port=5
  wires:
  In5/1 -> Out5/1
  In4/1 -> Out4/1
  In3/1 -> Out3/1
  In1/1 -> Out1/1
  In2/1 -> Out2/1
